simulink model "Lab1PartA4"  (R2016a)
settings: Solver=VariableStepAuto  StartTime=0.0  StopTime=20.0  RelTol=1e-3
settings Model: Creator=pzastawn  LastModifiedBy=pzastawn

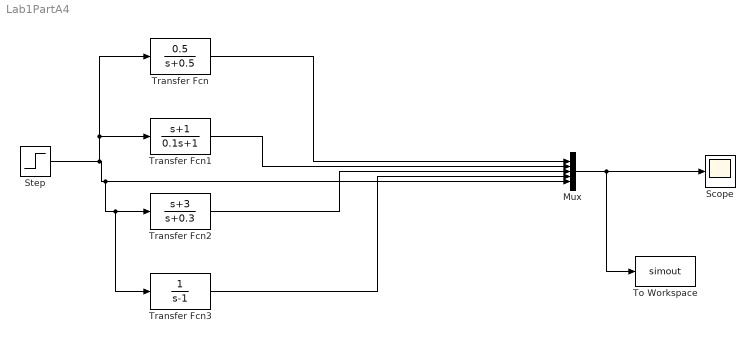
== system Lab1PartA4 ==
  Mux : Mux  Inputs=5
  Scope : Scope
  Step : Step  SampleTime=0
  To Workspace : ToWorkspace  VariableName=simout  SaveFormat=Timeseries  SampleTime=-1
  Transfer Fcn : TransferFcn  Numerator=[0.5]  Denominator=[1 0.5]
  Transfer Fcn1 : TransferFcn  Numerator=[1 1]  Denominator=[0.1 1]
  Transfer Fcn2 : TransferFcn  Numerator=[1 3]  Denominator=[1 0.3]
  Transfer Fcn3 : TransferFcn  Denominator=[1 -1]
  wires:
  Transfer Fcn/1 -> Mux/1
  Transfer Fcn1/1 -> Mux/2
  Transfer Fcn2/1 -> Mux/3
  Transfer Fcn3/1 -> Mux/4
  Step/1 -> Transfer Fcn1/1, Transfer Fcn/1, Transfer Fcn3/1, Transfer Fcn2/1, Mux/5
  Mux/1 -> To Workspace/1, Scope/1
